simulink library "PAYLOAD_MASTER"  (Simulink 8.8)
settings: Solver=ode45  StartTime=0.0  StopTime=10.0  RelTol=1e-3  EnableMultiTasking=on
libraries: cdsEpicsOut x123, cdsFilt x55, cdsTP x42, cdsFiltCtrl x33, cdsEpicsIn x31, cdsMuxMatrix x17, cdsEpicsBinIn x17, VIS_LIB x13, PAYLOAD_MASTER x13, cdsRms x8, simulink x6, cdsEpicsStringIn x6
(part 1 of 12)
settings Model: SuppressorTable=22 serialization::archive 11 0 3 0 0 0 11 0  Creator=controls  LastModifiedBy=controls

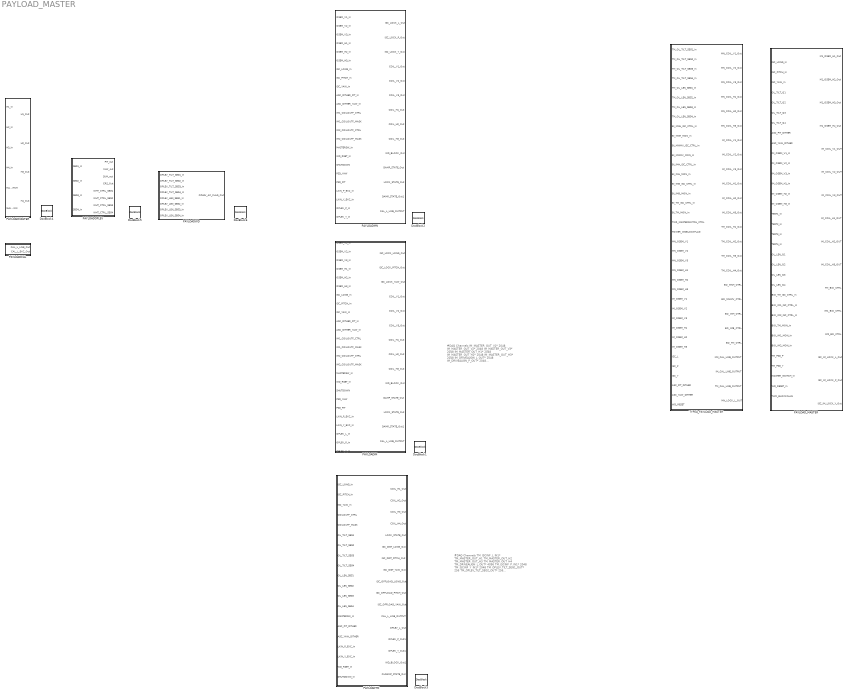
== system PAYLOAD_MASTER ==
  note: #DAQ Channels
      | IM_MASTER_OUT_V1* 2048
      | IM_MASTER_OUT_V2* 2048
      | IM_MASTER_OUT_V3* 2048
      | IM_MASTER_OUT_H1* 2048
      | IM_MASTER_OUT_H2* 2048
      | IM_MASTER_OUT_H3* 2048
      | IM_DRIVEALIGN_L_OUT* 2048
      | IM_DRIVEALIGN_P_OUT* 2048
      | IM_DRIVEALIGN_Y_OUT* 2048
      | IM_CAL_LINE_OUT* 512
      | IM_OLDAMP_P_OUT* 256
      | IM_OLDAMP_Y_OUT* 256
      | IM_OSEMINF_V1_OUT* 256
      | IM_OSEMINF_V2_OUT* 256
      | IM_OSEMINF_V3_OUT* 256
      | IM_OSEMINF_H1_OUT* 256
      | IM_OSEMINF_H2_OUT* 256
      | IM_OSEMINF_H3_OUT* 256
  note: #DAQ Channels
      | TM_ISCINF_L_IN1*
      | TM_MASTER_OUT_H1
      | TM_MASTER_OUT_H2
      | TM_MASTER_OUT_H3
      | TM_MASTER_OUT_H4
      |
      | TM_DRIVEALIGN_L_OUT* 4096
      |
      | TM_ISCINF_P_IN1* 2048
      | TM_ISCINF_Y_IN1* 2048
      |
      | TM_OPLEV_TILT_SEG1_OUT* 256
      | TM_OPLEV_TILT_SEG2_OUT* 256
      | TM_OPLEV_TILT_SEG3_OUT* 256
      | TM_OPLEV_TILT_SEG4_OUT* 256
      | TM_OPLEV_LEN_SEG1_OUT* 256
      | TM_OPLEV_LEN_SEG2_OUT* 256
      | TM_OPLEV_LEN_SEG3_OUT* 256
      | TM_OPLEV_LEN_SEG4_OUT* 256
      |
      | TM_OPLEV_TILT_PIT_OUT* 256
      | TM_OPLEV_TILT_YAW_OUT* 256
      | TM_OPLEV_TILT_SUM_OUT* 256
      | TM_OPLEV_LEN_PIT_OUT* 256
      | TM_OPLEV_LEN_YAW_OUT* 256
      | TM_OPLEV_LEN_SUM_OUT* 256
  DocBlock{1..6} (6 alike) : simulink/Model-Wide Utilities/DocBlock  DocumentType=Text
  PAYLOADCAL : Subsystem
  PAYLOADIM : Subsystem  Description=SIXOSEMSTAGE_FACE_MASTER
  PAYLOADMASTER : Subsystem
  PAYLOADMN : Subsystem  Description=SIXOSEMSTAGE_FACE_MASTER
  PAYLOADOPLEV : Subsystem
  PAYLOADTM : Subsystem
  PAYLOADWD : Subsystem
  PAYLOAD_MASTER : Subsystem  Description=This is for Type-B and Bp payloads.
      settings: AttributesFormatString=%<Description>
  TYPEA_PAYLOAD_MASTER : Subsystem  Description=This block is for Type-A payloads.

== system PAYLOAD_MASTER/PAYLOADCAL ==
  COSMON : cdsEpicsOut/Subsystem  Tag=cdsEpicsOutput  Description=|
      | Purpose:                                          
      | Output a FE signal to an EPICS channel.           
      |                                                   
      | Operation:                                        
      | Takes input value and passes it to EPICS record.  
      |                                                   
      | Usage:                                            
      | Name the part with the desired EPICS rrecord name.
      settings: AttributesFormatString=%<Tag>
  EXC : cdsEXC/Subsystem  Tag=Excitation
      settings: AttributesFormatString=%<Tag>
  EXCMON : cdsEpicsOut/Subsystem  Tag=cdsEpicsOutput  Description=|
      | Purpose:                                          
      | Output a FE signal to an EPICS channel.           
      |                                                   
      | Operation:                                        
      | Takes input value and passes it to EPICS record.  
      |                                                   
      | Usage:                                            
      | Name the part with the desired EPICS rrecord name.
      settings: AttributesFormatString=%<Tag>
  EXC_OUT : cdsTP/Subsystem  Tag=Test Point
      settings: AttributesFormatString=%<Tag>
  Ground2 : Ground
  LINE : cdsOscFixedPhase/Subsystem  Tag=cdsOscFixedPhase  Description=ADL=OSC.adl
      settings: AttributesFormatString=%<Tag>
  LINEMON : cdsEpicsOut/Subsystem  Tag=cdsEpicsOutput  Description=|
      | Purpose:                                          
      | Output a FE signal to an EPICS channel.           
      |                                                   
      | Operation:                                        
      | Takes input value and passes it to EPICS record.  
      |                                                   
      | Usage:                                            
      | Name the part with the desired EPICS rrecord name.
      settings: AttributesFormatString=%<Tag>
  LINE_OUT : cdsTP/Subsystem  Tag=Test Point
      settings: AttributesFormatString=%<Tag>
  SINMON : cdsEpicsOut/Subsystem  Tag=cdsEpicsOutput  Description=|
      | Purpose:                                          
      | Output a FE signal to an EPICS channel.           
      |                                                   
      | Operation:                                        
      | Takes input value and passes it to EPICS record.  
      |                                                   
      | Usage:                                            
      | Name the part with the desired EPICS rrecord name.
      settings: AttributesFormatString=%<Tag>
  Terminator : Terminator
  Terminator1 : Terminator
  CAL_L_LINE_Out : Outport
  CAL_L_EXC_Out : Outport  Port=2
  wires:
  LINEMON/1 -> CAL_L_LINE_Out/1, LINE_OUT/1
  SINMON/1 -> Terminator/1
  LINE/1 -> LINEMON/1
  LINE/2 -> SINMON/1
  COSMON/1 -> Terminator1/1
  LINE/3 -> COSMON/1
  Ground2/1 -> LINE/1
  EXCMON/1 -> CAL_L_EXC_Out/1
  EXC/1 -> EXC_OUT/1, EXCMON/1

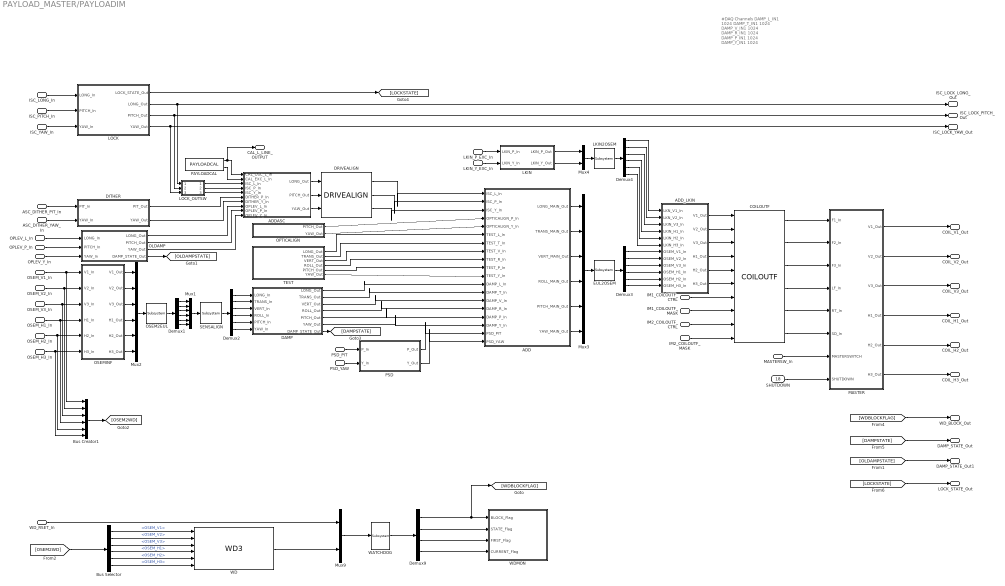
== system PAYLOAD_MASTER/PAYLOADIM ==
  note: #DAQ Channels
      | DAMP_L_IN1 1024
      | DAMP_T_IN1 1024
      | DAMP_V_IN1 1024
      | DAMP_R_IN1 1024
      | DAMP_P_IN1 1024
      | DAMP_Y_IN1 1024
  OSEM_V1_In : Inport
  OSEM_V2_In : Inport  Port=2
  OSEM_V3_In : Inport  Port=3
  OSEM_H1_In : Inport  Port=4
  OSEM_H2_In : Inport  Port=5
  OSEM_H3_In : Inport  Port=6
  ISC_LONG_In : Inport  Port=7
  ISC_PITCH_In : Inport  Port=8
  ISC_YAW_In : Inport  Port=9
  ASC_DITHER_PIT_In : Inport  Port=10
  ASC_DITHER_YAW_In : Inport  Port=11
  IM1_COILOUTF_CTRL : Inport  Port=12
  IM1_COILOUTF_MASK : Inport  Port=13
  IM2_COILOUTF_CTRL : Inport  Port=14
  IM2_COILOUTF_MASK : Inport  Port=15
  MASTERSW_In : Inport  Port=16
  WD_RSET_In : Inport  Port=17
  SHUTDOWN : Inport  Port=18
  PSD_YAW : Inport  Port=19
  PSD_PIT : Inport  Port=20
  LKIN_P_EXC_In : Inport  Port=21
  LKIN_Y_EXC_In : Inport  Port=22
  OPLEV_L_In : Inport  Port=23
  OPLEV_P_In : Inport  Port=24
  OPLEV_Y_In : Inport  Port=25
  ADD : Subsystem
  ADDASC : Subsystem
  ADD_LKIN : Subsystem
  Bus Creator1 : BusCreator  Inputs='OSEM_V1','OSEM_V2','OSEM_V3','OSEM_H1','OSEM_H2','OSEM_H3'
  Bus Selector : BusSelector  OutputSignals=OSEM_V1,OSEM_V2,OSEM_V3,OSEM_H1,OSEM_H2,OSEM_H3
  COILOUTF : SIXOSEM_F_COILOUTF_MASTER/COILOUTF
  DAMP : Subsystem
  DITHER : Subsystem
  DRIVEALIGN : VIS_LIB/DRIVEALIGN
  Demux{1..4} (4 alike) : Demux  Outputs=6
  Demux9 : Demux
  EUL2OSEM : cdsMuxMatrix/Subsystem  Tag=cdsMuxMatrix  Description=Any size matrix. Inputs and outputs must be connected using Mux and Demux parts.
      settings: AttributesFormatString=%<Tag>
  LKIN : Subsystem
  LKIN2OSEM : cdsMuxMatrix/Subsystem  Tag=cdsMuxMatrix  Description=Any size matrix. Inputs and outputs must be connected using Mux and Demux parts.
      settings: AttributesFormatString=%<Tag>
  LOCK : Subsystem
  LOCK_OUTSW : Subsystem
  MASTER : Subsystem
  Mux1 : Mux  Inputs=6
  Mux2 : Mux  Inputs=6
  Mux3 : Mux  Inputs=6
  Mux4 : Mux  Inputs=2
  Mux9 : Mux  Inputs=2
  OLDAMP : Subsystem
  OPTICALIGN : Subsystem
  OSEM2EUL : cdsMuxMatrix/Subsystem  Tag=cdsMuxMatrix  Description=Any size matrix. Inputs and outputs must be connected using Mux and Demux parts.
      settings: AttributesFormatString=%<Tag>
  OSEMINF : Subsystem
  PAYLOADCAL : PAYLOAD_MASTER/PAYLOADCAL
  PSD : Subsystem
  SENSALIGN : cdsMuxMatrix/Subsystem  Tag=cdsMuxMatrix  Description=Any size matrix. Inputs and outputs must be connected using Mux and Demux parts.
      settings: AttributesFormatString=%<Tag>
  TEST : Subsystem
  WATCHDOG : cdsFunctionCall/Subsystem  Tag=cdsFunctionCall  Description=inline OSEMWATCHDOG /opt/rtcds/userapps/release/vis/common/src/WATCHDOG.c
      settings: AttributesFormatString=%<Tag>\n%<Description>
  WD : VIS_LIB/WD3
  WDMON : Subsystem
  ISC_LOCK_LONG_Out : Outport
  ISC_LOCK_PITCH_Out : Outport  Port=2
  ISC_LOCK_YAW_Out : Outport  Port=3
  COIL_V1_Out : Outport  Port=4
  COIL_V2_Out : Outport  Port=5
  COIL_V3_Out : Outport  Port=6
  COIL_H1_Out : Outport  Port=7
  COIL_H2_Out : Outport  Port=8
  COIL_H3_Out : Outport  Port=9
  WD_BLOCK_Out : Outport  Port=10
  DAMP_STATE_Out : Outport  Port=11
  LOCK_STATE_Out : Outport  Port=12
  DAMP_STATE_Out1 : Outport  Port=13
  CAL_L_LINE_OUTPUT : Outport  Port=14
  wires:
  IM2_COILOUTF_MASK/1 -> COILOUTF/10
  IM2_COILOUTF_CTRL/1 -> COILOUTF/9
  LKIN_Y_EXC_In/1 -> LKIN/2(LKIN_Y_In)
  LKIN_P_EXC_In/1 -> LKIN/1(LKIN_P_In)
  DAMP/1(LONG_Out) -> ADD/12(DAMP_L_In)
  DAMP/2(TRANS_Out) -> ADD/13(DAMP_T_In)
  DAMP/3(VERT_Out) -> ADD/14(DAMP_V_In)
  DAMP/4(ROLL_Out) -> ADD/15(DAMP_R_In)
  DAMP/5(PITCH_Out) -> ADD/16(DAMP_P_In)
  DAMP/6(YAW_Out) -> ADD/17(DAMP_Y_In)
  TEST/1(LONG_Out) -> ADD/6(TEST_L_In)
  TEST/2(TRANS_Out) -> ADD/7(TEST_T_In)
  TEST/3(VERT_Out) -> ADD/8(TEST_V_In)
  TEST/4(ROLL_Out) -> ADD/9(TEST_R_In)
  TEST/5(PITCH_Out) -> ADD/10(TEST_P_In)
  TEST/6(YAW_Out) -> ADD/11(TEST_Y_In)
  OPTICALIGN/1(PITCH_Out) -> ADD/4(OPTICALIGN_P_In)
  OPTICALIGN/2(YAW_Out) -> ADD/5(OPTICALIGN_Y_In)
  ASC_DITHER_PIT_In/1 -> DITHER/1(PIT_In)
  ASC_DITHER_YAW_In/1 -> DITHER/2(YAW_In)
  ADDASC/3(YAW_Out) -> DRIVEALIGN/3
  ADDASC/2(PITCH_Out) -> DRIVEALIGN/2
  DRIVEALIGN/1 -> ADD/1(ISC_L_In)
  DRIVEALIGN/2 -> ADD/2(ISC_P_In)
  DRIVEALIGN/3 -> ADD/3(ISC_Y_In)
  LOCK/4(YAW_Out) -> LOCK_OUTSW/3(Y_In), ISC_LOCK_YAW_Out/1
  LOCK/3(PITCH_Out) -> LOCK_OUTSW/2(P_In), ISC_LOCK_PITCH_Out/1
  LOCK/2(LONG_Out) -> LOCK_OUTSW/1(L_In), ISC_LOCK_LONG_Out/1
  WD_RSET_In/1 -> Mux9/1
  WD/1 -> Mux9/2
  LKIN/2(LKIN_Y_Out) -> Mux4/2
  IM1_COILOUTF_CTRL/1 -> COILOUTF/7
  IM1_COILOUTF_MASK/1 -> COILOUTF/8
  MASTERSW_In/1 -> MASTER/7(MASTERSWITCH)
  Demux3/6 -> ADD_LKIN/12(OSEM_H3_In)
  Demux3/5 -> ADD_LKIN/11(OSEM_H2_In)
  Demux3/4 -> ADD_LKIN/10(OSEM_H1_In)
  Demux3/3 -> ADD_LKIN/9(OSEM_V3_In)
  Demux3/2 -> ADD_LKIN/8(OSEM_V2_In)
  Demux3/1 -> ADD_LKIN/7(OSEM_V1_In)
  Demux4/6 -> ADD_LKIN/6(LKIN_H3_In)
  Demux4/5 -> ADD_LKIN/5(LKIN_H2_In)
  Demux4/4 -> ADD_LKIN/4(LKIN_H1_In)
  Demux4/3 -> ADD_LKIN/3(LKIN_V3_In)
  Demux4/2 -> ADD_LKIN/2(LKN_V2_In)
  Demux4/1 -> ADD_LKIN/1(LKN_V1_In)
  ADD_LKIN/6(H3_Out) -> COILOUTF/6
  ADD_LKIN/5(H2_Out) -> COILOUTF/5
  ADD_LKIN/4(H1_Out) -> COILOUTF/4
  ADD_LKIN/3(V3_Out) -> COILOUTF/3
  ADD_LKIN/2(V2_Out) -> COILOUTF/2
  ADD_LKIN/1(V1_Out) -> COILOUTF/1
  Mux4/1 -> LKIN2OSEM/1
  LKIN2OSEM/1 -> Demux4/1
  LKIN/1(LKIN_P_Out) -> Mux4/1
  [LOCKSTATE] -> LOCK_STATE_Out/1
  LOCK/1(LOCK_STATE_Out) -> [LOCKSTATE]
  ADD/6(YAW_MAIN_Out) -> Mux3/6
  ADD/5(PITCH_MAIN_Out) -> Mux3/5
  ADD/4(ROLL_MAIN_Out) -> Mux3/4
  ADD/3(VERT_MAIN_Out) -> Mux3/3
  ADD/2(TRANS_MAIN_Out) -> Mux3/2
  ADD/1(LONG_MAIN_Out) -> Mux3/1
  [DAMPSTATE] -> DAMP_STATE_Out/1
  DAMP/7(DAMP_STATE_Out) -> [DAMPSTATE]
  [WDBLOCKFLAG] -> WD_BLOCK_Out/1
  Demux2/6 -> DAMP/6(YAW_In)
  Demux2/5 -> DAMP/5(PITCH_In)
  Demux2/4 -> DAMP/4(ROLL_In)
  Demux2/3 -> DAMP/3(VERT_In)
  Demux2/2 -> DAMP/2(TRANS_In)
  Demux2/1 -> DAMP/1(LONG_In)
  SHUTDOWN/1 -> MASTER/8(SHUTDOWN)
  OSEMINF/6(H3_Out) -> Mux2/6
  OSEMINF/5(H2_Out) -> Mux2/5
  OSEMINF/4(H1_Out) -> Mux2/4
  OSEMINF/3(V3_Out) -> Mux2/3
  OSEMINF/2(V2_Out) -> Mux2/2
  OSEMINF/1(V1_Out) -> Mux2/1
  OSEM_V1_In/1 -> OSEMINF/1(V1_In), Bus Creator1/1
  OSEM_V2_In/1 -> OSEMINF/2(V2_In), Bus Creator1/2
  OSEM_V3_In/1 -> OSEMINF/3(V3_In), Bus Creator1/3
  OSEM_H1_In/1 -> OSEMINF/4(H1_In), Bus Creator1/4
  OSEM_H2_In/1 -> OSEMINF/5(H2_In), Bus Creator1/5
  OSEM_H3_In/1 -> Bus Creator1/6, OSEMINF/6(H3_In)
  Mux2/1 -> OSEM2EUL/1
  ISC_LONG_In/1 -> LOCK/1(LONG_In)
  ISC_PITCH_In/1 -> LOCK/2(PITCH_In)
  ISC_YAW_In/1 -> LOCK/3(YAW_In)
  Bus Creator1/1 -> [OSEM2WD]
  [OSEM2WD] -> Bus Selector/1
  Bus Selector/1 -> WD/1  "<OSEM_V1>"
  Bus Selector/2 -> WD/2  "<OSEM_V2>"
  Bus Selector/3 -> WD/3  "<OSEM_V3>"
  Bus Selector/4 -> WD/4  "<OSEM_H1>"
  Bus Selector/5 -> WD/5  "<OSEM_H2>"
  Bus Selector/6 -> WD/6  "<OSEM_H3>"
  OSEM2EUL/1 -> Demux1/1
  Demux1/1 -> Mux1/1
  Demux1/2 -> Mux1/2
  Demux1/3 -> Mux1/3
  Demux1/4 -> Mux1/4
  Demux1/5 -> Mux1/5
  Demux1/6 -> Mux1/6
  Mux1/1 -> SENSALIGN/1
  SENSALIGN/1 -> Demux2/1
  MASTER/1(V1_Out) -> COIL_V1_Out/1
  MASTER/2(V2_Out) -> COIL_V2_Out/1
  MASTER/3(V3_Out) -> COIL_V3_Out/1
  MASTER/4(H1_Out) -> COIL_H1_Out/1
  MASTER/5(H2_Out) -> COIL_H2_Out/1
  MASTER/6(H3_Out) -> COIL_H3_Out/1
  Mux3/1 -> EUL2OSEM/1
  EUL2OSEM/1 -> Demux3/1
  Demux9/1 -> [WDBLOCKFLAG], WDMON/1(BLOCK_Flag)
  Demux9/2 -> WDMON/2(STATE_Flag)
  Demux9/3 -> WDMON/3(FIRST_Flag)
  Demux9/4 -> WDMON/4(CURRENT_Flag)
  COILOUTF/1 -> MASTER/1(F1_In)
  COILOUTF/2 -> MASTER/2(F2_In)
  COILOUTF/3 -> MASTER/3(F3_In)
  COILOUTF/4 -> MASTER/4(LF_In)
  COILOUTF/5 -> MASTER/5(RT_In)
  COILOUTF/6 -> MASTER/6(SD_In)
  Mux9/1 -> WATCHDOG/1
  WATCHDOG/1 -> Demux9/1
  PSD_PIT/1 -> PSD/1(P_In)
  PSD_YAW/1 -> PSD/2(Y_In)
  PSD/1(P_Out) -> ADD/18(PSD_PIT)
  PSD/2(Y_Out) -> ADD/19(PSD_YAW)
  ADDASC/1(LONG_Out) -> DRIVEALIGN/1
  DITHER/1(PIT_Out) -> ADDASC/6(DITHER_P_In)
  DITHER/2(YAW_Out) -> ADDASC/7(DITHER_Y_In)
  OLDAMP/1(LONG_Out) -> ADDASC/8(OPLEV_L_In)
  OLDAMP/2(PITCH_Out) -> ADDASC/9(OPLEV_P_In)
  LOCK_OUTSW/1(Out1) -> ADDASC/3(ISC_L_In)
  LOCK_OUTSW/2(Out2) -> ADDASC/4(ISC_P_In)
  LOCK_OUTSW/3(Out3) -> ADDASC/5(ISC_Y_In)
  [OLDAMPSTATE] -> DAMP_STATE_Out1/1
  PAYLOADCAL/2 -> ADDASC/2(CAL_EXC_L_In)
  PAYLOADCAL/1 -> ADDASC/1(CAL_OSC_L_In), CAL_L_LINE_OUTPUT/1
  OPLEV_P_In/1 -> OLDAMP/2(PITCH_In)
  OPLEV_Y_In/1 -> OLDAMP/3(YAW_In)
  OPLEV_L_In/1 -> OLDAMP/1(LONG_In)
  OLDAMP/4(DAMP_STATE_Out) -> [OLDAMPSTATE]
  OLDAMP/3(YAW_Out) -> ADDASC/10(OPLEV_Y_In)

== system PAYLOAD_MASTER/PAYLOADMASTER ==
  note: If second input (WDFLAG) is not equal to zero,
      | then pass out first argument (Constant 0 -- Block Output),
      | otherwise pass out third arguement (Constant 1 -- Pass Output)
  note: WDFLAG is 0 (zero) if OK,
      | Non-zero if BAD
  H1_In : Inport
  H2_In : Inport  Port=2
  H3_In : Inport  Port=3
  H4_In : Inport  Port=4
  MASTERSWITCH : Inport  Port=5
  SHUTDOWN : Inport  Port=6
  Add : Sum  Inputs=-+
  Constant1 : Constant
  OUT_H{1..4} (4 alike) : cdsTP/Subsystem  Tag=Test Point
      settings: AttributesFormatString=%<Tag>
  OUT_H1MON : cdsEpicsOut/Subsystem  Tag=cdsEpicsOutput  Description=|
      | Purpose:                                          
      | Output a FE signal to an EPICS channel.           
      |                                                   
      | Operation:                                        
      | Takes input value and passes it to EPICS record.  
      |                                                   
      | Usage:                                            
      | Name the part with the desired EPICS rrecord name.
      settings: AttributesFormatString=%<Tag>
  OUT_H2MON : cdsEpicsOut/Subsystem  Tag=cdsEpicsOutput  Description=|
      | Purpose:                                          
      | Output a FE signal to an EPICS channel.           
      |                                                   
      | Operation:                                        
      | Takes input value and passes it to EPICS record.  
      |                                                   
      | Usage:                                            
      | Name the part with the desired EPICS rrecord name.
      settings: AttributesFormatString=%<Tag>
  OUT_H3MON : cdsEpicsOut/Subsystem  Tag=cdsEpicsOutput  Description=|
      | Purpose:                                          
      | Output a FE signal to an EPICS channel.           
      |                                                   
      | Operation:                                        
      | Takes input value and passes it to EPICS record.  
      |                                                   
      | Usage:                                            
      | Name the part with the desired EPICS rrecord name.
      settings: AttributesFormatString=%<Tag>
  OUT_H4MON : cdsEpicsOut/Subsystem  Tag=cdsEpicsOutput  Description=|
      | Purpose:                                          
      | Output a FE signal to an EPICS channel.           
      |                                                   
      | Operation:                                        
      | Takes input value and passes it to EPICS record.  
      |                                                   
      | Usage:                                            
      | Name the part with the desired EPICS rrecord name.
      settings: AttributesFormatString=%<Tag>
  PWD_H{1..4} (4 alike) : cdsTP/Subsystem  Tag=Test Point
      settings: AttributesFormatString=%<Tag>
  PWD_H1MON : cdsEpicsOut/Subsystem  Tag=cdsEpicsOutput  Description=|
      | Purpose:                                          
      | Output a FE signal to an EPICS channel.           
      |                                                   
      | Operation:                                        
      | Takes input value and passes it to EPICS record.  
      |                                                   
      | Usage:                                            
      | Name the part with the desired EPICS rrecord name.
      settings: AttributesFormatString=%<Tag>
  PWD_H2MON : cdsEpicsOut/Subsystem  Tag=cdsEpicsOutput  Description=|
      | Purpose:                                          
      | Output a FE signal to an EPICS channel.           
      |                                                   
      | Operation:                                        
      | Takes input value and passes it to EPICS record.  
      |                                                   
      | Usage:                                            
      | Name the part with the desired EPICS rrecord name.
      settings: AttributesFormatString=%<Tag>
  PWD_H3MON : cdsEpicsOut/Subsystem  Tag=cdsEpicsOutput  Description=|
      | Purpose:                                          
      | Output a FE signal to an EPICS channel.           
      |                                                   
      | Operation:                                        
      | Takes input value and passes it to EPICS record.  
      |                                                   
      | Usage:                                            
      | Name the part with the desired EPICS rrecord name.
      settings: AttributesFormatString=%<Tag>
  PWD_H4MON : cdsEpicsOut/Subsystem  Tag=cdsEpicsOutput  Description=|
      | Purpose:                                          
      | Output a FE signal to an EPICS channel.           
      |                                                   
      | Operation:                                        
      | Takes input value and passes it to EPICS record.  
      |                                                   
      | Usage:                                            
      | Name the part with the desired EPICS rrecord name.
      settings: AttributesFormatString=%<Tag>
  P_MS_H{1..4} (4 alike) : Product  RndMeth=Zero
  P_WD_H{1..4} (4 alike) : Product  RndMeth=Zero
  SWITCHMON : cdsEpicsOut/Subsystem  Tag=cdsEpicsOutput  Description=|
      | Purpose:                                          
      | Output a FE signal to an EPICS channel.           
      |                                                   
      | Operation:                                        
      | Takes input value and passes it to EPICS record.  
      |                                                   
      | Usage:                                            
      | Name the part with the desired EPICS rrecord name.
      settings: AttributesFormatString=%<Tag>
  Terminator2 : Terminator
  H1_Out : Outport
  H2_Out : Outport  Port=2
  H3_Out : Outport  Port=3
  H4_Out : Outport  Port=4
  wires:
  Add/1 -> P_WD_H1/2, P_WD_H2/2, P_WD_H3/2, P_WD_H4/2
  PWD_H4MON/1 -> P_WD_H4/1
  PWD_H3MON/1 -> P_WD_H3/1
  PWD_H2MON/1 -> P_WD_H2/1
  PWD_H1MON/1 -> P_WD_H1/1
  H1_In/1 -> P_MS_H1/2
  H2_In/1 -> P_MS_H2/2
  H3_In/1 -> P_MS_H3/2
  H4_In/1 -> P_MS_H4/2
  MASTERSWITCH/1 -> P_MS_H4/1, P_MS_H3/1, P_MS_H2/1, P_MS_H1/1, SWITCHMON/1
  OUT_H2MON/1 -> H2_Out/1
  OUT_H1MON/1 -> H1_Out/1
  OUT_H3MON/1 -> H3_Out/1
  OUT_H4MON/1 -> H4_Out/1
  P_MS_H1/1 -> PWD_H1MON/1, PWD_H1/1
  P_MS_H2/1 -> PWD_H2MON/1, PWD_H2/1
  P_MS_H3/1 -> PWD_H3MON/1, PWD_H3/1
  P_MS_H4/1 -> PWD_H4MON/1, PWD_H4/1
  P_WD_H1/1 -> OUT_H1MON/1, OUT_H1/1
  P_WD_H2/1 -> OUT_H2MON/1, OUT_H2/1
  P_WD_H3/1 -> OUT_H3MON/1, OUT_H3/1
  P_WD_H4/1 -> OUT_H4MON/1, OUT_H4/1
  SWITCHMON/1 -> Terminator2/1
  SHUTDOWN/1 -> Add/1
  Constant1/1 -> Add/2

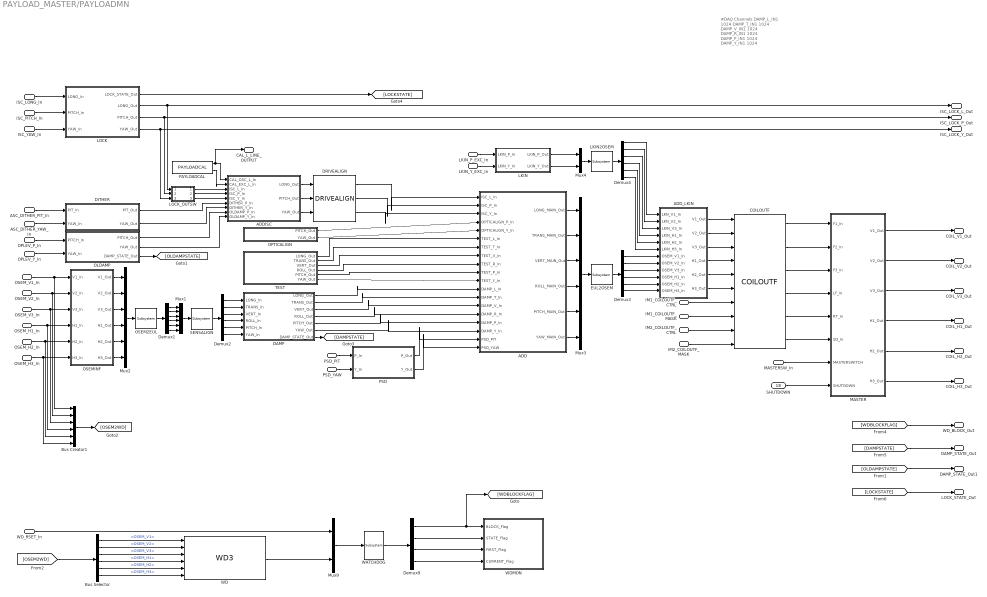
== system PAYLOAD_MASTER/PAYLOADMN ==
  note: #DAQ Channels
      | DAMP_L_IN1 1024
      | DAMP_T_IN1 1024
      | DAMP_V_IN1 1024
      | DAMP_R_IN1 1024
      | DAMP_P_IN1 1024
      | DAMP_Y_IN1 1024
  OSEM_V1_In : Inport
  OSEM_V2_In : Inport  Port=2
  OSEM_V3_In : Inport  Port=3
  OSEM_H1_In : Inport  Port=4
  OSEM_H2_In : Inport  Port=5
  OSEM_H3_In : Inport  Port=6
  ISC_LONG_In : Inport  Port=7
  ISC_PITCH_In : Inport  Port=8
  ISC_YAW_In : Inport  Port=9
  ASC_DITHER_PIT_In : Inport  Port=10
  ASC_DITHER_YAW_In : Inport  Port=11
  IM1_COILOUTF_CTRL : Inport  Port=12
  IM1_COILOUTF_MASK : Inport  Port=13
  IM2_COILOUTF_CTRL : Inport  Port=14
  IM2_COILOUTF_MASK : Inport  Port=15
  MASTERSW_In : Inport  Port=16
  WD_RSET_In : Inport  Port=17
  SHUTDOWN : Inport  Port=18
  PSD_YAW : Inport  Port=19
  PSD_PIT : Inport  Port=20
  LKIN_P_EXC_In : Inport  Port=21
  LKIN_Y_EXC_In : Inport  Port=22
  OPLEV_P_In : Inport  Port=23
  OPLEV_Y_In : Inport  Port=24
  ADD : Subsystem
  ADDISC : Subsystem
  ADD_LKIN : Subsystem
  Bus Creator1 : BusCreator  Inputs='OSEM_V1','OSEM_V2','OSEM_V3','OSEM_H1','OSEM_H2','OSEM_H3'
  Bus Selector : BusSelector  OutputSignals=OSEM_V1,OSEM_V2,OSEM_V3,OSEM_H1,OSEM_H2,OSEM_H3
  COILOUTF : SIXOSEM_F_COILOUTF_MASTER/COILOUTF
  DAMP : Subsystem
  DITHER : Subsystem
  DRIVEALIGN : VIS_LIB/DRIVEALIGN
  Demux{1..4} (4 alike) : Demux  Outputs=6
  Demux9 : Demux
  EUL2OSEM : cdsMuxMatrix/Subsystem  Tag=cdsMuxMatrix  Description=Any size matrix. Inputs and outputs must be connected using Mux and Demux parts.
      settings: AttributesFormatString=%<Tag>
  LKIN : Subsystem
  LKIN2OSEM : cdsMuxMatrix/Subsystem  Tag=cdsMuxMatrix  Description=Any size matrix. Inputs and outputs must be connected using Mux and Demux parts.
      settings: AttributesFormatString=%<Tag>
  LOCK : Subsystem
  LOCK_OUTSW : Subsystem
  MASTER : Subsystem
  Mux1 : Mux  Inputs=6
  Mux2 : Mux  Inputs=6
  Mux3 : Mux  Inputs=6
  Mux4 : Mux  Inputs=2
  Mux9 : Mux  Inputs=2
  OLDAMP : Subsystem
  OPTICALIGN : Subsystem
  OSEM2EUL : cdsMuxMatrix/Subsystem  Tag=cdsMuxMatrix  Description=Any size matrix. Inputs and outputs must be connected using Mux and Demux parts.
      settings: AttributesFormatString=%<Tag>
  OSEMINF : Subsystem
  PAYLOADCAL : PAYLOAD_MASTER/PAYLOADCAL
  PSD : Subsystem
  SENSALIGN : cdsMuxMatrix/Subsystem  Tag=cdsMuxMatrix  Description=Any size matrix. Inputs and outputs must be connected using Mux and Demux parts.
      settings: AttributesFormatString=%<Tag>
  TEST : Subsystem
  WATCHDOG : cdsFunctionCall/Subsystem  Tag=cdsFunctionCall  Description=inline OSEMWATCHDOG /opt/rtcds/userapps/release/vis/common/src/WATCHDOG.c
      settings: AttributesFormatString=%<Tag>\n%<Description>
  WD : VIS_LIB/WD3
  WDMON : Subsystem
  ISC_LOCK_L_Out : Outport
  ISC_LOCK_P_Out : Outport  Port=2
  ISC_LOCK_Y_Out : Outport  Port=3
  COIL_V1_Out : Outport  Port=4
  COIL_V2_Out : Outport  Port=5
  COIL_V3_Out : Outport  Port=6
  COIL_H1_Out : Outport  Port=7
  COIL_H2_Out : Outport  Port=8
  COIL_H3_Out : Outport  Port=9
  WD_BLOCK_Out : Outport  Port=10
  DAMP_STATE_Out : Outport  Port=11
  LOCK_STATE_Out : Outport  Port=12
  DAMP_STATE_Out1 : Outport  Port=13
  CAL_L_LINE_OUTPUT : Outport  Port=14
  wires:
  IM2_COILOUTF_MASK/1 -> COILOUTF/10
  IM2_COILOUTF_CTRL/1 -> COILOUTF/9
  LKIN_Y_EXC_In/1 -> LKIN/2(LKIN_Y_In)
  LKIN_P_EXC_In/1 -> LKIN/1(LKIN_P_In)
  DAMP/1(LONG_Out) -> ADD/12(DAMP_L_In)
  DAMP/2(TRANS_Out) -> ADD/13(DAMP_T_In)
  DAMP/3(VERT_Out) -> ADD/14(DAMP_V_In)
  DAMP/4(ROLL_Out) -> ADD/15(DAMP_R_In)
  DAMP/5(PITCH_Out) -> ADD/16(DAMP_P_In)
  DAMP/6(YAW_Out) -> ADD/17(DAMP_Y_In)
  TEST/1(LONG_Out) -> ADD/6(TEST_L_In)
  TEST/2(TRANS_Out) -> ADD/7(TEST_T_In)
  TEST/3(VERT_Out) -> ADD/8(TEST_V_In)
  TEST/4(ROLL_Out) -> ADD/9(TEST_R_In)
  TEST/5(PITCH_Out) -> ADD/10(TEST_P_In)
  TEST/6(YAW_Out) -> ADD/11(TEST_Y_In)
  OPTICALIGN/1(PITCH_Out) -> ADD/4(OPTICALIGN_P_In)
  OPTICALIGN/2(YAW_Out) -> ADD/5(OPTICALIGN_Y_In)
  ASC_DITHER_PIT_In/1 -> DITHER/1(PIT_In)
  ASC_DITHER_YAW_In/1 -> DITHER/2(YAW_In)
  ADDISC/3(YAW_Out) -> DRIVEALIGN/3
  ADDISC/2(PITCH_Out) -> DRIVEALIGN/2
  DRIVEALIGN/1 -> ADD/1(ISC_L_In)
  DRIVEALIGN/2 -> ADD/2(ISC_P_In)
  DRIVEALIGN/3 -> ADD/3(ISC_Y_In)
  LOCK/4(YAW_Out) -> LOCK_OUTSW/3(Y_In), ISC_LOCK_Y_Out/1
  LOCK/3(PITCH_Out) -> LOCK_OUTSW/2(P_In), ISC_LOCK_P_Out/1
  LOCK/2(LONG_Out) -> LOCK_OUTSW/1(L_In), ISC_LOCK_L_Out/1
  WD_RSET_In/1 -> Mux9/1
  WD/1 -> Mux9/2
  LKIN/2(LKIN_Y_Out) -> Mux4/2
  IM1_COILOUTF_CTRL/1 -> COILOUTF/7
  IM1_COILOUTF_MASK/1 -> COILOUTF/8
  MASTERSW_In/1 -> MASTER/7(MASTERSWITCH)
  Demux3/6 -> ADD_LKIN/12(OSEM_H3_In)
  Demux3/5 -> ADD_LKIN/11(OSEM_H2_In)
  Demux3/4 -> ADD_LKIN/10(OSEM_H1_In)
  Demux3/3 -> ADD_LKIN/9(OSEM_V3_In)
  Demux3/2 -> ADD_LKIN/8(OSEM_V2_In)
  Demux3/1 -> ADD_LKIN/7(OSEM_V1_In)
  Demux4/6 -> ADD_LKIN/6(LKIN_H3_In)
  Demux4/5 -> ADD_LKIN/5(LKIN_H2_In)
  Demux4/4 -> ADD_LKIN/4(LKIN_H1_In)
  Demux4/3 -> ADD_LKIN/3(LKIN_V3_In)
  Demux4/2 -> ADD_LKIN/2(LKN_V2_In)
  Demux4/1 -> ADD_LKIN/1(LKN_V1_In)
  ADD_LKIN/6(H3_Out) -> COILOUTF/6
  ADD_LKIN/5(H2_Out) -> COILOUTF/5
  ADD_LKIN/4(H1_Out) -> COILOUTF/4
  ADD_LKIN/3(V3_Out) -> COILOUTF/3
  ADD_LKIN/2(V2_Out) -> COILOUTF/2
  ADD_LKIN/1(V1_Out) -> COILOUTF/1
  Mux4/1 -> LKIN2OSEM/1
  LKIN2OSEM/1 -> Demux4/1
  LKIN/1(LKIN_P_Out) -> Mux4/1
  [LOCKSTATE] -> LOCK_STATE_Out/1
  LOCK/1(LOCK_STATE_Out) -> [LOCKSTATE]
  ADD/6(YAW_MAIN_Out) -> Mux3/6
  ADD/5(PITCH_MAIN_Out) -> Mux3/5
  ADD/4(ROLL_MAIN_Out) -> Mux3/4
  ADD/3(VERT_MAIN_Out) -> Mux3/3
  ADD/2(TRANS_MAIN_Out) -> Mux3/2
  ADD/1(LONG_MAIN_Out) -> Mux3/1
  [DAMPSTATE] -> DAMP_STATE_Out/1
  DAMP/7(DAMP_STATE_Out) -> [DAMPSTATE]
  [WDBLOCKFLAG] -> WD_BLOCK_Out/1
  Demux2/6 -> DAMP/6(YAW_In)
  Demux2/5 -> DAMP/5(PITCH_In)
  Demux2/4 -> DAMP/4(ROLL_In)
  Demux2/3 -> DAMP/3(VERT_In)
  Demux2/2 -> DAMP/2(TRANS_In)
  Demux2/1 -> DAMP/1(LONG_In)
  SHUTDOWN/1 -> MASTER/8(SHUTDOWN)
  OSEMINF/6(H3_Out) -> Mux2/6
  OSEMINF/5(H2_Out) -> Mux2/5
  OSEMINF/4(H1_Out) -> Mux2/4
  OSEMINF/3(V3_Out) -> Mux2/3
  OSEMINF/2(V2_Out) -> Mux2/2
  OSEMINF/1(V1_Out) -> Mux2/1
  OSEM_V1_In/1 -> OSEMINF/1(V1_In), Bus Creator1/1
  OSEM_V2_In/1 -> OSEMINF/2(V2_In), Bus Creator1/2
  OSEM_V3_In/1 -> OSEMINF/3(V3_In), Bus Creator1/3
  OSEM_H1_In/1 -> OSEMINF/4(H1_In), Bus Creator1/4
  OSEM_H2_In/1 -> OSEMINF/5(H2_In), Bus Creator1/5
  OSEM_H3_In/1 -> Bus Creator1/6, OSEMINF/6(H3_In)
  Mux2/1 -> OSEM2EUL/1
  ISC_LONG_In/1 -> LOCK/1(LONG_In)
  ISC_PITCH_In/1 -> LOCK/2(PITCH_In)
  ISC_YAW_In/1 -> LOCK/3(YAW_In)
  Bus Creator1/1 -> [OSEM2WD]
  [OSEM2WD] -> Bus Selector/1
  Bus Selector/1 -> WD/1  "<OSEM_V1>"
  Bus Selector/2 -> WD/2  "<OSEM_V2>"
  Bus Selector/3 -> WD/3  "<OSEM_V3>"
  Bus Selector/4 -> WD/4  "<OSEM_H1>"
  Bus Selector/5 -> WD/5  "<OSEM_H2>"
  Bus Selector/6 -> WD/6  "<OSEM_H3>"
  OSEM2EUL/1 -> Demux1/1
  Demux1/1 -> Mux1/1
  Demux1/2 -> Mux1/2
  Demux1/3 -> Mux1/3
  Demux1/4 -> Mux1/4
  Demux1/5 -> Mux1/5
  Demux1/6 -> Mux1/6
  Mux1/1 -> SENSALIGN/1
  SENSALIGN/1 -> Demux2/1
  MASTER/1(V1_Out) -> COIL_V1_Out/1
  MASTER/2(V2_Out) -> COIL_V2_Out/1
  MASTER/3(V3_Out) -> COIL_V3_Out/1
  MASTER/4(H1_Out) -> COIL_H1_Out/1
  MASTER/5(H2_Out) -> COIL_H2_Out/1
  MASTER/6(H3_Out) -> COIL_H3_Out/1
  Mux3/1 -> EUL2OSEM/1
  EUL2OSEM/1 -> Demux3/1
  Demux9/1 -> [WDBLOCKFLAG], WDMON/1(BLOCK_Flag)
  Demux9/2 -> WDMON/2(STATE_Flag)
  Demux9/3 -> WDMON/3(FIRST_Flag)
  Demux9/4 -> WDMON/4(CURRENT_Flag)
  COILOUTF/1 -> MASTER/1(F1_In)
  COILOUTF/2 -> MASTER/2(F2_In)
  COILOUTF/3 -> MASTER/3(F3_In)
  COILOUTF/4 -> MASTER/4(LF_In)
  COILOUTF/5 -> MASTER/5(RT_In)
  COILOUTF/6 -> MASTER/6(SD_In)
  Mux9/1 -> WATCHDOG/1
  WATCHDOG/1 -> Demux9/1
  PSD_PIT/1 -> PSD/1(P_In)
  PSD_YAW/1 -> PSD/2(Y_In)
  PSD/1(P_Out) -> ADD/18(PSD_PIT)
  PSD/2(Y_Out) -> ADD/19(PSD_YAW)
  OPLEV_P_In/1 -> OLDAMP/1(PITCH_In)
  OPLEV_Y_In/1 -> OLDAMP/2(YAW_In)
  ADDISC/1(LONG_Out) -> DRIVEALIGN/1
  DITHER/1(PIT_Out) -> ADDISC/6(DITHER_P_In)
  DITHER/2(YAW_Out) -> ADDISC/7(DITHER_Y_In)
  OLDAMP/1(PITCH_Out) -> ADDISC/8(OLDAMP_P_In)
  OLDAMP/2(YAW_Out) -> ADDISC/9(OLDAMP_Y_In)
  LOCK_OUTSW/1(Out1) -> ADDISC/3(ISC_L_In)
  LOCK_OUTSW/2(Out2) -> ADDISC/4(ISC_P_In)
  LOCK_OUTSW/3(Out3) -> ADDISC/5(ISC_Y_In)
  OLDAMP/3(DAMP_STATE_Out) -> [OLDAMPSTATE]
  [OLDAMPSTATE] -> DAMP_STATE_Out1/1
  PAYLOADCAL/2 -> ADDISC/2(CAL_EXC_L_In)
  PAYLOADCAL/1 -> CAL_L_LINE_OUTPUT/1, ADDISC/1(CAL_OSC_L_In)
